simulink model "threephase_converter_IGBT"  (R2024a)
settings: Solver=VariableStepAuto  StartTime=0.0  StopTime=10  RelTol=1e-3
libraries: spsIGBTDiodeLib x6, spsVoltageMeasurementLib x4, spsACVoltageSourceLib x3, spsSeriesRLCBranchLib x1, sps_lib x1
settings Model: Creator=farza  LastModifiedBy=farza

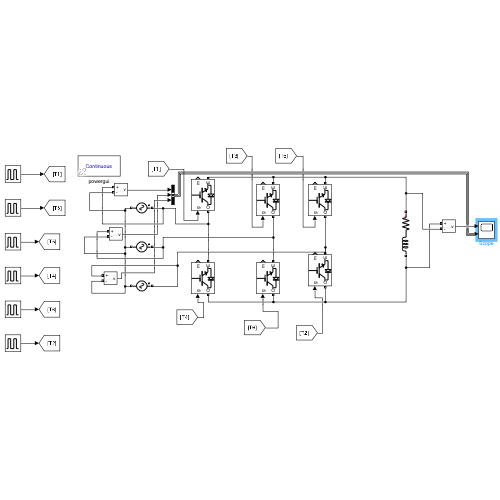
[thumbnail: Simulink's stored preview of the top-level diagram]
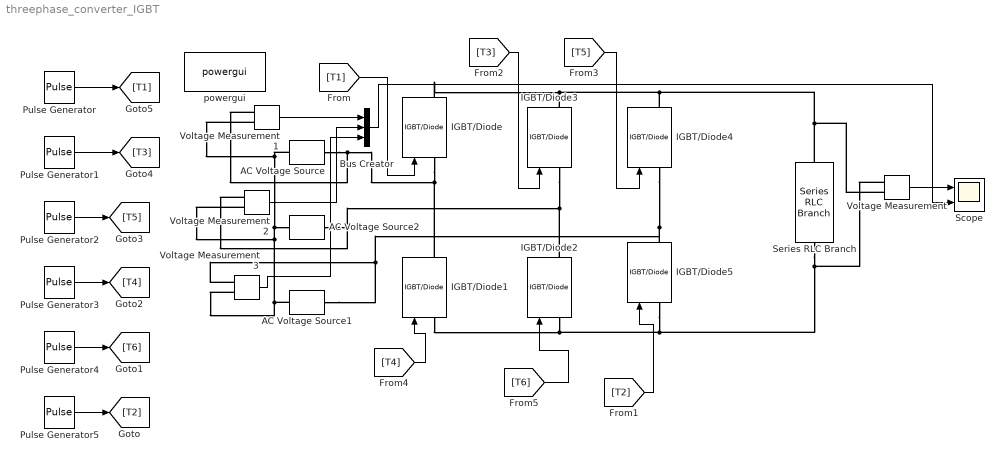
== system threephase_converter_IGBT ==
  AC Voltage Source : spsACVoltageSourceLib/AC Voltage Source  Amplitude=230*1.414  Phase=0  Frequency=50  SampleTime=0  Measurements=Voltage  BusType=swing  Pref=10e3  Qref=0  Qmin=-inf  Qmax=+inf
  AC Voltage Source1 : spsACVoltageSourceLib/AC Voltage Source  Amplitude=230*1.414  Phase=-240  Frequency=50  SampleTime=0  Measurements=Voltage  BusType=swing  Pref=10e3  Qref=0  Qmin=-inf  Qmax=+inf
  AC Voltage Source2 : spsACVoltageSourceLib/AC Voltage Source  Amplitude=230*1.414  Phase=-120  Frequency=50  SampleTime=0  Measurements=Voltage  BusType=swing  Pref=10e3  Qref=0  Qmin=-inf  Qmax=+inf
  Bus Creator : BusCreator  Inputs=3
  IGBT/Diode{,1..5} (6 alike) : spsIGBTDiodeLib/IGBT//Diode  Ron=1e-3  Rs=1e5  Cs=inf  Measurements=on
  Pulse Generator : DiscretePulseGenerator  PulseType=Time based  Period=0.02  PulseWidth=120*100/360  PhaseDelay=90*(0.02/360)
  Pulse Generator1 : DiscretePulseGenerator  PulseType=Time based  Period=0.02  PulseWidth=120*100/360  PhaseDelay=210*(0.02/360)
  Pulse Generator2 : DiscretePulseGenerator  PulseType=Time based  Period=0.02  PulseWidth=120*100/360  PhaseDelay=330*(0.02/360)
  Pulse Generator3 : DiscretePulseGenerator  PulseType=Time based  Period=0.02  PulseWidth=120*100/360  PhaseDelay=270*(0.02/360)
  Pulse Generator4 : DiscretePulseGenerator  PulseType=Time based  Period=0.02  PulseWidth=120*100/360  PhaseDelay=390*(0.02/360)
  Pulse Generator5 : DiscretePulseGenerator  PulseType=Time based  Period=0.02  PulseWidth=120*100/360  PhaseDelay=150*(0.02/360)
  Scope : Scope  NumInputPorts=2
  Series RLC Branch : spsSeriesRLCBranchLib/Series RLC Branch  LConnTagsString=__new0  RConnTagsString=__new0  BranchType=RL  Resistance=10  Inductance=2.5  SetiL0=on  InitialCurrent=0  Capacitance=1e-6  Setx0=off  InitialVoltage=0  Measurements=Branch voltage and current
  Voltage Measurement{,1..3} (4 alike) : spsVoltageMeasurementLib/Voltage Measurement  PhasorSimulation=off  OutputType=Complex  PSBequivalent=0
  powergui : sps_lib/powergui  Priority=1  SimulationMode=Continuous  SampleTime=50e-6  frequency=60  Iterations=50  frequencyindice=50  Pbase=100e6  ErrMax=1e-4  UnitsV=kV  UnitsW=MW  buscounter=0  FunctionMessages=off  echomessages=off  EnableUseOfTLC=off  CurrentSourceSwitches=off  DisableSnubberDevices=off  DisableRonSwitches=off  DisableVfSwitches=off  DisplayEquations=off  AutomaticDiscreteSolvers=off  SolverType=Tustin/Backward Euler (TBE)  Interpol=off  ExternalGateDelay=off  methode=off  Ts=100  x0status=blocks  SPID=on  SwTol=0  HookPort=off  NonlinearTolerance=1e-4  nMaxIteration=100  ContinueOnMaxIteration=off  RestoreLinks=warning  ResistiveCurrentMeasurement=off  Frange=[0:2:500]  Ylog=off  Xlog=on  ShowGrid=off  save=off  variable=ZData  structure=0  ZoomFFT=off  StartTime=0.0  cycles=1  DisplayStyle=1  fundamental=60  FreqAxis=off  MaxFrequency=1000  frequencyindicesteady=1  RmsSteady=1  display=off
  wires:
  [T1] -> IGBT/Diode/1
  [T3] -> IGBT/Diode3/1
  [T5] -> IGBT/Diode4/1
  [T4] -> IGBT/Diode1/1
  [T6] -> IGBT/Diode2/1
  [T2] -> IGBT/Diode5/1
  Pulse Generator/1 -> [T1]
  Pulse Generator1/1 -> [T3]
  Pulse Generator2/1 -> [T5]
  Pulse Generator3/1 -> [T4]
  Pulse Generator4/1 -> [T6]
  Pulse Generator5/1 -> [T2]
  Voltage Measurement/1 -> Scope/1
  Voltage Measurement1/1 -> Bus Creator/1
  Voltage Measurement2/1 -> Bus Creator/2
  Voltage Measurement3/1 -> Bus Creator/3
  Bus Creator/1 -> Scope/2
  connections:
  Voltage Measurement1/LConn1 -- AC Voltage Source/RConn1 -- IGBT/Diode1/RConn1 -- IGBT/Diode/LConn1
  Voltage Measurement2/LConn1 -- AC Voltage Source2/RConn1 -- IGBT/Diode3/LConn1 -- IGBT/Diode2/RConn1
  Voltage Measurement/LConn2 -- Series RLC Branch/LConn1 -- IGBT/Diode4/RConn1 -- IGBT/Diode3/RConn1 -- IGBT/Diode/RConn1
  AC Voltage Source1/RConn1 -- Voltage Measurement3/LConn1 -- IGBT/Diode5/RConn1 -- IGBT/Diode4/LConn1
  Voltage Measurement/LConn1 -- Series RLC Branch/RConn1 -- IGBT/Diode5/LConn1 -- IGBT/Diode2/LConn1 -- IGBT/Diode1/LConn1
  AC Voltage Source/LConn1 -- Voltage Measurement1/LConn2 -- Voltage Measurement2/LConn2 -- Voltage Measurement3/LConn2 -- AC Voltage Source1/LConn1 -- AC Voltage Source2/LConn1
